simulink model "TAULab3"  (R2014b)
settings: Solver=ode45  StartTime=0.0  StopTime=10.0  RelTol=1e-3
settings Model: Creator=kiril_000  LastModifiedBy=kiril_000

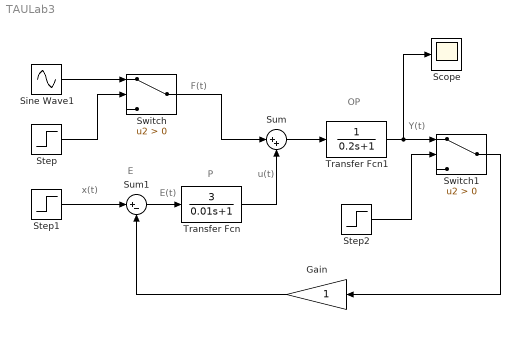
== system TAULab3 ==
  note: Y(t)
  note: u(t)
  note: F(t)
  note: OP
  note: P
  note: E(t)
  note: Е
  note: x(t)
  Gain : Gain
  Scope : Scope
      settings: TimeRange=10  YMin=0  YMax=3.5
  Sine Wave1 : Sin  Frequency=10  SampleTime=0
  Step : Step  SampleTime=2
  Step1 : Step  SampleTime=0
  Step2 : Step  SampleTime=6
  Sum : Sum  Inputs=|++
  Sum1 : Sum  Inputs=|+-
  Switch : Switch  Criteria=u2 > Threshold
  Switch1 : Switch  Criteria=u2 > Threshold
  Transfer Fcn : TransferFcn  Numerator=[3]  Denominator=[0.01 1]
  Transfer Fcn1 : TransferFcn  Denominator=[0.2 1]
  wires:
  Sine Wave1/1 -> Switch/1
  Step/1 -> Switch/2
  Switch/1 -> Sum/1
  Transfer Fcn/1 -> Sum/2
  Sum/1 -> Transfer Fcn1/1
  Step2/1 -> Switch1/2
  Switch1/1 -> Gain/1
  Gain/1 -> Sum1/2
  Sum1/1 -> Transfer Fcn/1
  Step1/1 -> Sum1/1
  Transfer Fcn1/1 -> Scope/1, Switch1/1
